simulink model "dynamic_calib"  (Simulink 8.8)
settings: Solver=FixedStepDiscrete  StartTime=0.0  StopTime=20.0  FixedStep=CONFIG.Ts  RelTol=1e-3  EnableMultiTasking=on
values from neighbouring files (symbols this model uses):
  calibDelta = newOffsets*pi/180    [kinematic_calib.m]
libraries: WBToolboxLibrary x13
settings Model: SuppressorTable=22 serialization::archive 11 0 3 0 0 0 11 0  Creator=gabri  LastModifiedBy=leo
settings DataIOCC: SignalLoggingSaveFormat=Dataset
settings DebuggingCC: UnderspecifiedInitializationDetection=Simplified  MergeDetectMultiDrivingBlocksExec=error  SolverPrmCheckMsg=warning  FcnCallInpInsideContextMsg=error  StateNameClashWarn=none
settings GRTTargetCC: CombineOutputUpdateFcns=on  GRTInterface=off
settings ConfigComp: CovSFcnEnable=off

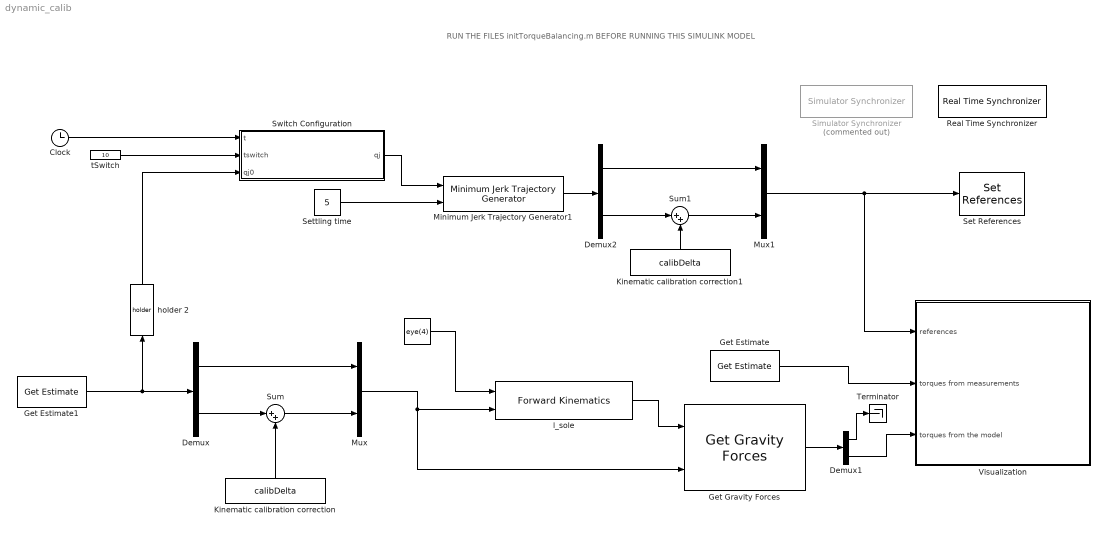
== system dynamic_calib ==
  note: RUN THE FILES initTorqueBalancing.m BEFORE RUNNING THIS SIMULINK MODEL
  " " : Constant  Value=eye(4)
  Clock : Clock
  Demux : Demux  Outputs=[13;12]
  Demux1 : Demux  Outputs=[6;25]
  Demux2 : Demux  Outputs=[13;12]
  Get Estimate : WBToolboxLibrary/wholeBodyStates/Get Estimate  estimateType=Joints Torque  robotName=WBT_robotName  localName=WBT_modelName  wbiFile=WBT_wbiFilename  wbiList=WBT_wbiList
  Get Estimate1 : WBToolboxLibrary/wholeBodyStates/Get Estimate  estimateType=Joints Position  robotName=WBT_robotName  localName=WBT_modelName  wbiFile=WBT_wbiFilename  wbiList=WBT_wbiList
  Get Gravity Forces : WBToolboxLibrary/wholeBodyModel/Dynamics/Get Gravity Forces  robotName=WBT_robotName  localName=WBT_modelName  wbiFile=WBT_wbiFilename  wbiList=WBT_wbiList  explicitGravity=off
  Kinematic calibration correction : Constant  Value=calibDelta
  Kinematic calibration correction1 : Constant  Value=calibDelta
  Minimum Jerk Trajectory Generator1 : WBToolboxLibrary/Utilities/Minimum Jerk Trajectory Generator  externalSettlingTime=on  settlingTime=1  sampleTime=CONFIG.Ts  resetOnSettlingTime=off  firstDerivatives=off  secondDerivatives=off  explicitInitialValue=off
  Mux : Mux  Inputs=2
  Mux1 : Mux  Inputs=2
  Real Time Synchronizer : WBToolboxLibrary/Utilities/Real Time Synchronizer  period=0.01
  Set References : WBToolboxLibrary/wholeBodyActuators/Set References  controlType=Position Direct  fullOrSubControl=Full  controlledJoints=''  robotName=WBT_robotName  localName=WBT_modelName  wbiFile=WBT_wbiFilename  wbiList=WBT_wbiList
  Settling time : Constant  Value=5
  Simulator Synchronizer : WBToolboxLibrary/Utilities/Simulator Synchronizer  Commented=on  period=0.01  serverPortName='/clock/rpc'  clientPortName='/WBT_synchronizer/rpc:o'
  Sum : Sum  Inputs=|++
  Sum1 : Sum  Inputs=|++
  Switch Configuration : MATLAB Function  TreatAsAtomicUnit=on
  Terminator : Terminator
  Visualization : Subsystem
  holder 2 : WBToolboxLibrary/Utilities/holder 
  l_sole : WBToolboxLibrary/wholeBodyModel/Kinematics/Forward Kinematics  frameName='Waist'  robotName=WBT_robotName  localName=WBT_modelName  wbiFile=WBT_wbiFilename  wbiList=WBT_wbiList
  tSwitch : Constant  Value=10
  wires:
  l_sole/1 -> Get Gravity Forces/1
  Kinematic calibration correction/1 -> Sum/2
  Get Estimate/1 -> Visualization/2(torques from measurements)
  Get Estimate1/1 -> Demux/1, holder 2/1
  Demux/2 -> Sum/1
  Demux/1 -> Mux/1
  Mux/1 -> l_sole/2, Get Gravity Forces/2
  Sum/1 -> Mux/2
  Get Gravity Forces/1 -> Demux1/1
  Demux1/2 -> Visualization/3(torques from the model)
  Demux1/1 -> Terminator/1
  Switch Configuration/1(qj) -> Minimum Jerk Trajectory Generator1/1
  Settling time/1 -> Minimum Jerk Trajectory Generator1/2
  Clock/1 -> Switch Configuration/1(t)
  tSwitch/1 -> Switch Configuration/2(tswitch)
  Kinematic calibration correction1/1 -> Sum1/2
  Minimum Jerk Trajectory Generator1/1 -> Demux2/1
  Demux2/2 -> Sum1/1
  Demux2/1 -> Mux1/1
  Sum1/1 -> Mux1/2
  Mux1/1 -> Visualization/1(references), Set References/1
  " "/1 -> l_sole/1
  holder 2/1 -> Switch Configuration/3(qj0)

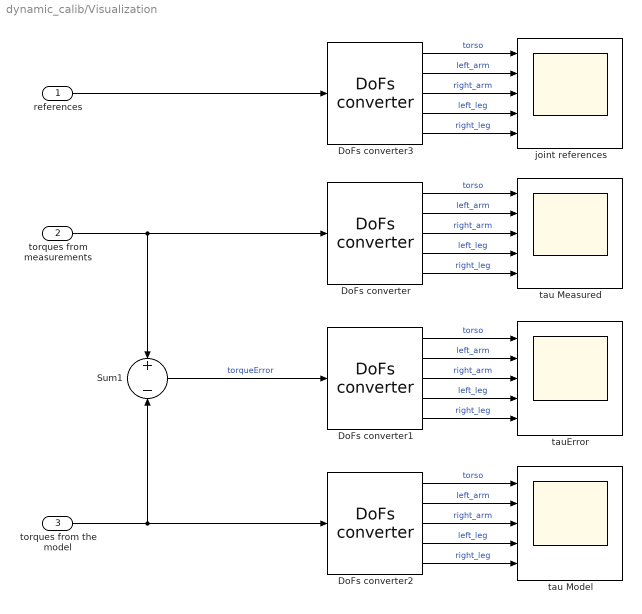
== system dynamic_calib/Visualization ==
  references : Inport
  torques from measurements : Inport  Port=2
  torques from the model : Inport  Port=3
  DoFs converter{,1..3} (4 alike) : WBToolboxLibrary/Utilities/DoFs converter  yarp2WBIOption=From WBI to YARP  robotName=WBT_robotName  localName=WBT_modelName  wbiFile=WBT_wbiFilename  wbiList=WBT_wbiList
  Sum1 : Sum  Inputs=+-
  joint references : Scope  NumInputPorts=5
  tau Measured : Scope  NumInputPorts=5
  tau Model : Scope  NumInputPorts=5
  tauError : Scope  NumInputPorts=5
  wires:
  DoFs converter2/3 -> tau Model/3  "right_arm"
  torques from the model/1 -> DoFs converter2/1, Sum1/2
  DoFs converter/4 -> tau Measured/4  "left_leg"
  DoFs converter/3 -> tau Measured/3  "right_arm"
  DoFs converter1/5 -> tauError/5  "right_leg"
  DoFs converter1/1 -> tauError/1  "torso"
  DoFs converter1/2 -> tauError/2  "left_arm"
  DoFs converter1/4 -> tauError/4  "left_leg"
  DoFs converter1/3 -> tauError/3  "right_arm"
  Sum1/1 -> DoFs converter1/1  "torqueError"
  DoFs converter2/5 -> tau Model/5  "right_leg"
  DoFs converter2/1 -> tau Model/1  "torso"
  DoFs converter2/2 -> tau Model/2  "left_arm"
  DoFs converter2/4 -> tau Model/4  "left_leg"
  torques from measurements/1 -> DoFs converter/1, Sum1/1
  DoFs converter/5 -> tau Measured/5  "right_leg"
  DoFs converter/1 -> tau Measured/1  "torso"
  DoFs converter/2 -> tau Measured/2  "left_arm"
  DoFs converter3/4 -> joint references/4  "left_leg"
  DoFs converter3/3 -> joint references/3  "right_arm"
  references/1 -> DoFs converter3/1
  DoFs converter3/5 -> joint references/5  "right_leg"
  DoFs converter3/1 -> joint references/1  "torso"
  DoFs converter3/2 -> joint references/2  "left_arm"

== matlab function Switch Configuration ==
  data: t input double; qj output double; tswitch input double; qj0 input double
function qj = changeConfigFCN(t,tswitch,qj0)

qj = changeConfig(t,tswitch,qj0);

end
